simulink model "simulink_only"  (R2020b)
settings: Solver=VariableStepAuto  StartTime=0.0  StopTime=inf  RelTol=1e-3
settings Model: Creator=Rick  LastModifiedBy=rick

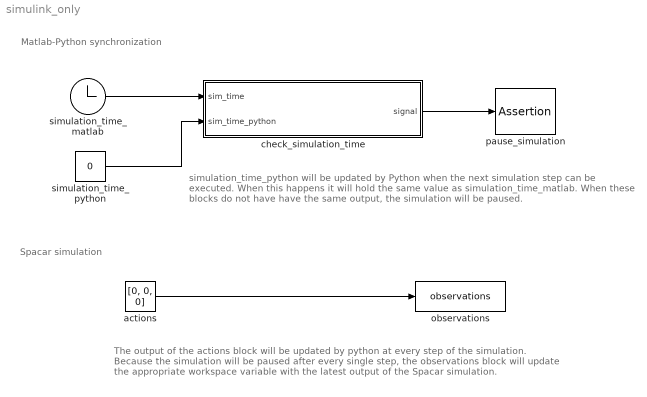
== system simulink_only ==
  note: The output of the actions block will be updated by python at every step of the simulation. Because the simulation will be paused after every single step, the observations block will update the appropriate workspace variable with the latest output of the Spacar simulation.
  note: simulation_time_python will be updated by Python when the next simulation step can be executed. When this happens it will hold the same value as simulation_time_matlab. When these blocks do not have have the same output, the simulation will be paused.
  note: Spacar simulation
  note: Matlab-Python synchronization
  actions : Constant  Value=[0, 0, 0]
  check_simulation_time : MATLAB Function  TreatAsAtomicUnit=on
  observations : ToWorkspace  VariableName=observations  SampleTime=-1
      settings: MaxDataPoints=1
  pause_simulation : Assertion  AssertionFailFcn=set_param(bdroot, 'SimulationCommand', 'pause')  StopWhenAssertionFail=off
  simulation_time_matlab : Clock
  simulation_time_python : Constant  Value=0
  wires:
  actions/1 -> observations/1
  simulation_time_matlab/1 -> check_simulation_time/1(sim_time)
  simulation_time_python/1 -> check_simulation_time/2(sim_time_python)
  check_simulation_time/1(signal) -> pause_simulation/1

== matlab function simulink_only/check_simulation_time ==
  data: sim_time input; sim_time_python input; signal output
function signal = assert_input(sim_time, sim_time_python)
    if sim_time > sim_time_python
        signal = 0; % pause sim until python let's it continue
    else if sim_time == sim_time_python
        signal = 1; % good to go
    else
        signal = 0;
        disp("Warning: Matlab' simulation is lagging behind Python.")
    end
end
